simulink model "lqr_controller"  (R2020b)
settings: Solver=VariableStepAuto  StartTime=0.0  StopTime=10.0  RelTol=1e-3
values from neighbouring files (symbols this model uses):
  A = [0 1 0 0 ... (first row only)    [simulation.m]
  B = [0; 1/M; 0; 1/(M*L)]    [simulation.m]
  C = [1 0 0 0]    [simulation.m]
  K = lqr(sys,Q,R)    [simulation.m]
settings Model: Creator=Ghost  LastModifiedBy=Ghost

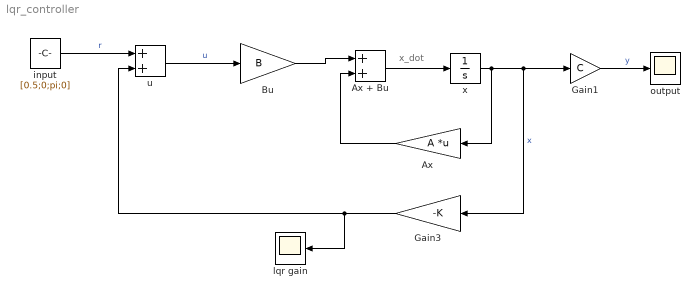
== system lqr_controller ==
  note: x_dot
  Ax : Gain  Gain=A  Multiplication=Matrix(K*u) (u vector)
  Ax + Bu : Sum
  Bu : Gain  Gain=B
  Gain1 : Gain  Gain=C
  Gain3 : Gain  Gain=-K
  input : Constant  Value=[0.5;0;pi;0]
  lqr gain : Scope
  output : Scope
  u : Sum
  x : Integrator
  wires:
  Bu/1 -> Ax + Bu/1
  Ax + Bu/1 -> x/1
  Gain1/1 -> output/1  "y"
  x/1 -> Ax/1, Gain3/1, Gain1/1  "x"
  Ax/1 -> Ax + Bu/2
  Gain3/1 -> u/2, lqr gain/1
  input/1 -> u/1  "r"
  u/1 -> Bu/1  "u"
